simulink model "gtcs_math_v2"  (R2022b)
settings: Solver=VariableStepAuto  StartTime=0.0  StopTime=10  RelTol=1e-3
undefined symbols (not defined in the file or in its folder): B_load, B_motor, B_reducer, GearRatio, J_load, J_motor, J_reducer, ke, kt, L_motor, R_motor
libraries: slpidlib x1, simulink x1
settings Model: DataDictionary=gtcs_math_v1.sldd  Creator=yusuf.ogut  LastModifiedBy=Yusuf
settings ModelReferenceCC: EnableRefExpFcnMdlSchedulingChecks=on

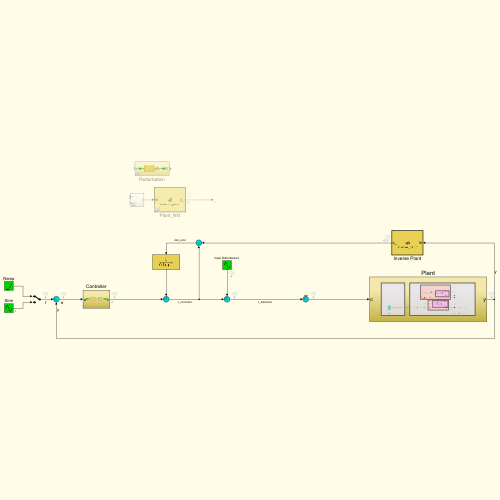
[thumbnail: Simulink's stored preview of the top-level diagram]
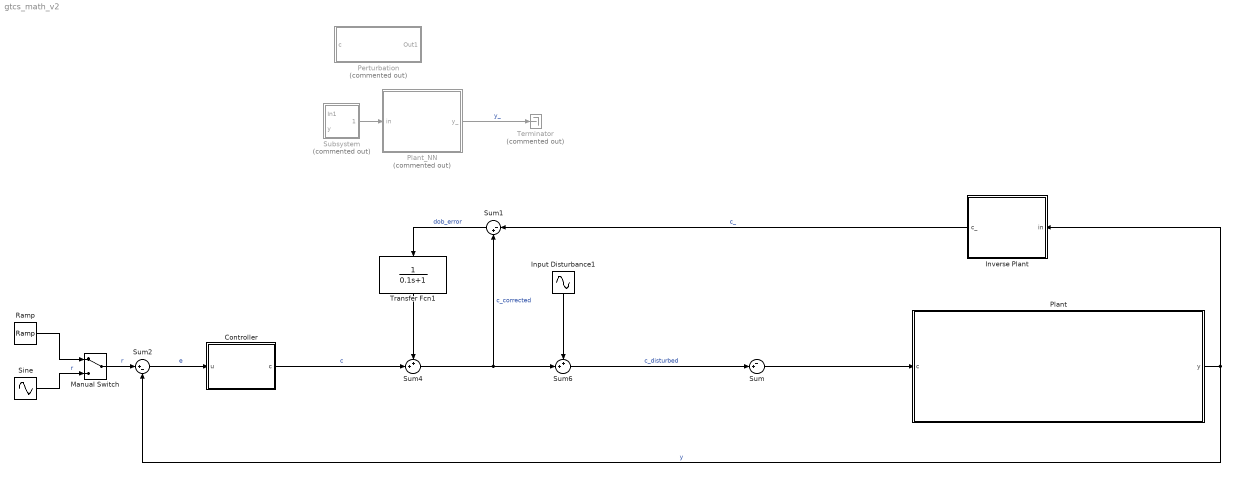
== system gtcs_math_v2 ==
  Controller : Subsystem
  Input Disturbance1 : Sin  SampleTime=0
  Inverse Plant : MATLAB Function  TreatAsAtomicUnit=on
  Manual Switch : ManualSwitch
  Perturbation : Subsystem  Commented=on
  Plant : Subsystem
  Plant_NN : MATLAB Function  Commented=on  TreatAsAtomicUnit=on
  Ramp : simulink/Sources/Ramp  slope=30  start=0  InitialOutput=0
  Sine : Sin  Amplitude=400  SampleTime=0
  Subsystem : Subsystem  Commented=on
  Sum : Sum  Inputs=-+|
  Sum1 : Sum  Inputs=|-+
  Sum2 : Sum  Inputs=|+-
  Sum4 : Sum  Inputs=++|
  Sum6 : Sum  Inputs=++|
  Terminator : Terminator  Commented=on
  Transfer Fcn1 : TransferFcn  Denominator=[0.1 1]
  wires:
  Plant/1(y) -> Inverse Plant/1(in), Sum2/2  "y"
  Sum2/1 -> Controller/1(u)  "e"
  Plant_NN/1(y_) -> Terminator/1  "y_"
  Sum/1 -> Plant/1(c)
  Sum6/1 -> Sum/2  "c_disturbed"
  Sine/1 -> Manual Switch/2  "r"
  Ramp/1 -> Manual Switch/1
  Manual Switch/1 -> Sum2/1  "r"
  Subsystem/1(Out1) -> Plant_NN/1(in)
  Controller/1(c) -> Sum4/2  "c"
  Sum4/1 -> Sum6/2, Sum1/2  "c_corrected"
  Input Disturbance1/1 -> Sum6/1
  Inverse Plant/1(c_) -> Sum1/1  "c_"
  Sum1/1 -> Transfer Fcn1/1  "dob_error"
  Transfer Fcn1/1 -> Sum4/1

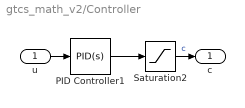
== system gtcs_math_v2/Controller ==
  u : Inport
  PID Controller1 : slpidlib/PID Controller  Controller=PID  Form=Parallel  TimeDomain=Continuous-time  UseExternalTs=off  SampleTime=-1  IntegratorMethod=Forward Euler  FilterMethod=Forward Euler  ControllerParametersSource=internal  P=1  I=0.12  UseKiTs=off  D=0  N=100  UseFilter=on  TunerSelectOption=Transfer Function Based (PID Tuner App)  InitialConditionSource=internal  InitialConditionForIntegrator=0  InitialConditionForFilter=0  DifferentiatorICPrevScaledInput=0  ExternalReset=none  TrackingMode=off  Kt=1  LimitOutput=off  SatLimitsSource=internal  UpperSaturationLimit=inf  LowerSaturationLimit=-inf  LinearizeAsGain=on  AntiWindupMode=none  Kb=1  LimitIntegrator=off  UpperIntegratorSaturationLimit=inf  LowerIntegratorSaturationLimit=-inf  POutMin=[]  POutMax=[]  IOutMin=[]  IOutMax=[]  DOutMin=[]  DOutMax=[]  NOutMin=[]  NOutMax=[]  SumOutMin=[]  SumOutMax=[]  SaturationOutMin=[]  SaturationOutMax=[]  PParamMin=[]  PParamMax=[]  IParamMin=[]  IParamMax=[]  DParamMin=[]  DParamMax=[]  NParamMin=[]  NParamMax=[]  KbParamMin=[]  KbParamMax=[]  KtParamMin=[]  KtParamMax=[]  KbOutMin=[]  KbOutMax=[]  KtOutMin=[]  KtOutMax=[]  IntegratorOutMin=[]  IntegratorOutMax=[]  FilterOutMin=[]  FilterOutMax=[]  SumI1OutMin=[]  SumI1OutMax=[]  SumI2OutMin=[]  SumI2OutMax=[]  SumI3OutMin=[]  SumI3OutMax=[]  SumI4OutMin=[]  SumI4OutMax=[]  SumDOutMin=[]  SumDOutMax=[]  DifferentiatorOutMin=[]  DifferentiatorOutMax=[]  FilterDiffOutCoefMin=[]  FilterDiffOutCoefMax=[]  ReciprocalOutMin=[]  ReciprocalOutMax=[]  SumDenOutMin=[]  SumDenOutMax=[]  SumNumOutMin=[]  SumNumOutMax=[]  DivideOutMin=[]  DivideOutMax=[]  UdiffTsProdOutMin=[]  UdiffTsProdOutMax=[]  NTsProdOutMin=[]  NTsProdOutMax=[]  UintegralTsProdOutMin=[]  UintegralTsProdOutMax=[]  UngainTsProdOutMin=[]  UngainTsProdOutMax=[]  ClampingZeroOutDataTypeStr=Inherit: Inherit via back propagation  ClampingZeroOutMin=[]  ClampingZeroOutMax=[]  FilterDenConstantOutDataTypeStr=Inherit: Inherit via back propagation  FilterDenConstantOutMin=[]  FilterDenConstantOutMax=[]  PCopyOutDataTypeStr=Inherit: Inherit via back propagation  PCopyOutMin=[]  PCopyOutMax=[]  NCopyOutDataTypeStr=Inherit: Inherit via back propagation  NCopyOutMin=[]  NCopyOutMax=[]  IntegratorContinuousStateAttributes=''  IntegratorStateMustResolveToSignalObject=off  IntegratorRTWStateStorageClass=Auto  FilterContinuousStateAttributes=''  FilterStateMustResolveToSignalObject=off  FilterRTWStateStorageClass=Auto  ParallelPVariant=InternalParameters  IdealPVariant=Disabled  IVariant=InternalParameters  DVariant=InternalParameters  IntegratorVariant=Continuous  SatVariant=Disabled  AWVariant=Passthrough  PCopyVariant=Disabled  TRVariant=Disabled  FdbkBlocksVariant=Forward  IdealPFdbkVariant=Disabled  SatFdbkVariant=Disabled  DerivativeFilterVariant=ContFilter  NVariant=InternalParameters  NCopyVariant=Disabled  FilterICVariant=InternalICsFilter  IntegratorICVariant=InternalICs  ExternalResetVariant=Disabled  TRSumVariant=Passthrough  SumFdbkVariant=Disabled  SumVariant=Sum_PID  TsampFilterVariant=InternalTs  TsampNgainVariant=Passthrough  TsampIntegralVariant=Passthrough  ExternalSaturationOutDataTypeStr=Inherit: Same as second input
  Saturation2 : Saturate  UpperLimit=28  LowerLimit=-28
  c : Outport
  wires:
  Saturation2/1 -> c/1  "c"
  PID Controller1/1 -> Saturation2/1
  u/1 -> PID Controller1/1

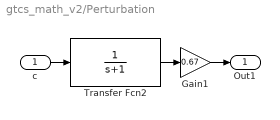
== system gtcs_math_v2/Perturbation ==
  c : Inport
  Gain1 : Gain  Gain=0.67
  Transfer Fcn2 : TransferFcn  Denominator=[1 1]
  Out1 : Outport
  wires:
  Gain1/1 -> Out1/1
  c/1 -> Transfer Fcn2/1
  Transfer Fcn2/1 -> Gain1/1

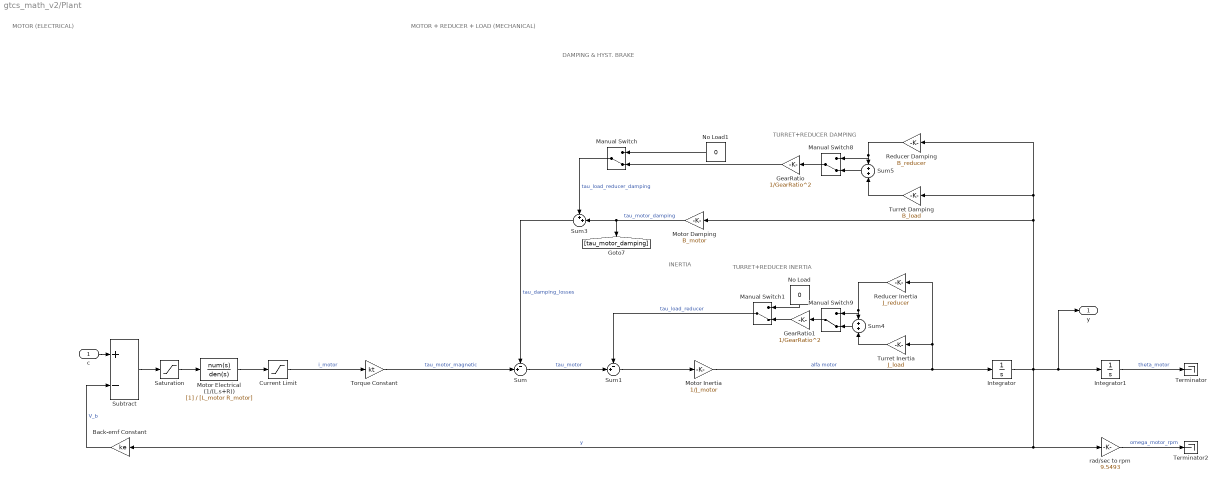
== system gtcs_math_v2/Plant ==
  note: TURRET+REDUCER INERTIA
  note: TURRET+REDUCER DAMPING
  note: DAMPING & HYST. BRAKE
  note: INERTIA
  note: MOTOR (ELECTRICAL)
  note: MOTOR + REDUCER + LOAD (MECHANICAL)
  c : Inport
  Back-emf Constant : Gain  Gain=ke
  Current Limit : Saturate  UpperLimit=80  LowerLimit=-80
  GearRatio : Gain  Gain=1/GearRatio^2
  GearRatio1 : Gain  Gain=1/GearRatio^2
  Integrator : Integrator
  Integrator1 : Integrator
  Manual Switch{,1,8..9} (4 alike) : ManualSwitch  CurrentSetting=0
  Motor Damping : Gain  Gain=B_motor
  Motor Electrical (1/(L.s+R)) : TransferFcn  Denominator=[L_motor R_motor]
  Motor Inertia : Gain  Gain=1/J_motor
  No Load : Constant  Value=0
  No Load1 : Constant  Value=0
  Reducer Damping : Gain  Gain=B_reducer
  Reducer Inertia : Gain  Gain=J_reducer
  Saturation : Saturate  UpperLimit=28  LowerLimit=-28
  Subtract : Sum  Inputs=+-
  Sum : Sum  Inputs=-+|
  Sum1 : Sum  Inputs=-+|
  Sum3 : Sum  Inputs=++|
  Sum4 : Sum
  Sum5 : Sum
  Terminator : Terminator
  Terminator2 : Terminator
  Torque Constant : Gain  Gain=kt
  Turret Damping : Gain  Gain=B_load
  Turret Inertia : Gain  Gain=J_load
  rad/sec to rpm : Gain  Gain=9.5493
  y : Outport
  wires:
  No Load/1 -> Manual Switch1/1
  Turret Damping/1 -> Sum5/2
  Reducer Inertia/1 -> Manual Switch9/1, Sum4/1
  GearRatio1/1 -> Manual Switch1/2
  Torque Constant/1 -> Sum/2  "tau_motor_magnetic"
  Manual Switch/1 -> Sum3/1  "tau_load_reducer_damping"
  Integrator/1 -> y/1, Integrator1/1, rad/sec to rpm/1, Back-emf Constant/1, Turret Damping/1, Reducer Damping/1, Motor Damping/1  "y"
  Current Limit/1 -> Torque Constant/1  "i_motor"
  No Load1/1 -> Manual Switch/1
  Manual Switch9/1 -> GearRatio1/1
  Sum3/1 -> Sum/1  "tau_damping_losses"
  Motor Inertia/1 -> Integrator/1, Turret Inertia/1, Reducer Inertia/1  "alfa motor"
  Sum4/1 -> Manual Switch9/2
  Sum1/1 -> Motor Inertia/1
  Manual Switch1/1 -> Sum1/1  "tau_load_reducer"
  GearRatio/1 -> Manual Switch/2
  Integrator1/1 -> Terminator/1  "theta_motor"
  Turret Inertia/1 -> Sum4/2
  Manual Switch8/1 -> GearRatio/1
  Reducer Damping/1 -> Manual Switch8/1, Sum5/1
  Sum/1 -> Sum1/2  "tau_motor"
  Motor Damping/1 -> [tau_motor_damping], Sum3/2  "tau_motor_damping"
  Sum5/1 -> Manual Switch8/2
  Saturation/1 -> Motor Electrical (1/(L.s+R))/1
  Back-emf Constant/1 -> Subtract/2  "V_b"
  c/1 -> Subtract/1
  rad/sec to rpm/1 -> Terminator2/1  "omega_motor_rpm"
  Motor Electrical (1/(L.s+R))/1 -> Current Limit/1
  Subtract/1 -> Saturation/1

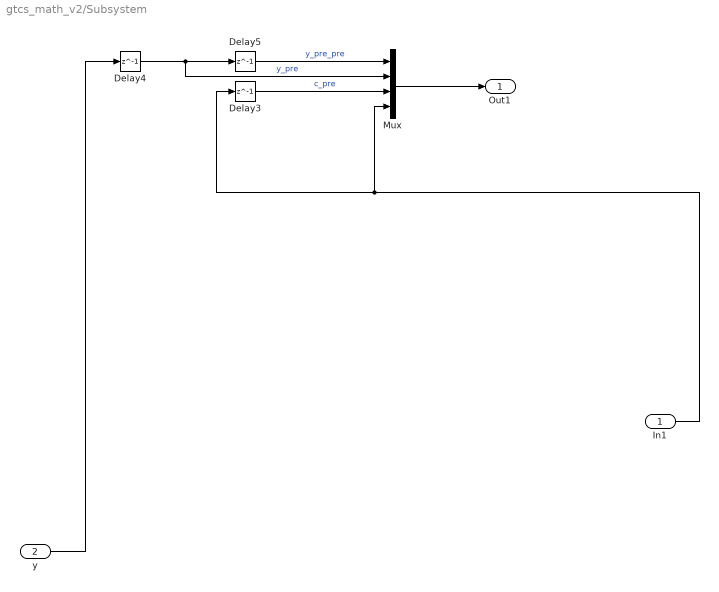
== system gtcs_math_v2/Subsystem ==
  In1 : Inport
  y : Inport  Port=2
  Delay3 : Delay  DelayLength=1  SampleTime=0.01
  Delay4 : Delay  DelayLength=1  SampleTime=0.01
  Delay5 : Delay  DelayLength=1  SampleTime=0.01
  Mux : Mux
  Out1 : Outport
  wires:
  In1/1 -> Mux/4, Delay3/1
  Delay4/1 -> Delay5/1, Mux/2  "y_pre"
  Delay3/1 -> Mux/3  "c_pre"
  Mux/1 -> Out1/1
  Delay5/1 -> Mux/1  "y_pre_pre"
  y/1 -> Delay4/1

== matlab function gtcs_math_v2/Inverse Plant ==
  data: in input; c_ output
function c_ = inverse_plant(in)
    y_ =  0.0534; r_ = 16.0258;
    c__ = 1.2811; r__ = 384.4721;
    input_training = (in - c__)/r__;
    Phi = [ -0.7229   -0.1132         0         0
            -0.7229   -0.1132         0         0
            -0.7229   -0.1132         0         0
            -0.4882   -0.4882   -0.4882   -0.1223];
    BIAS = -.1;
    % FORWARD PASS:
    NUM_INP = 1; NUM_HID = 3;
    input_vector = [input_training;BIAS];
    S1 = Phi(1:NUM_HID,1:NUM_INP+1)*input_vector;
    O1 = tanh(S1);
    S2 = Phi(NUM_HID+1:end,1:NUM_HID+1)*[O1;BIAS];
    c_ = S2*r_+y_;
end

== matlab function gtcs_math_v2/Plant_NN ==
  data: in input; y_ output
function y_ = forward_pass(in)
    c_sf_i_4 = 24.3519;     r_sf_i_4 = 3.6481;
    c_sf_i_3 = 14;          r_sf_i_3 = 14;
    c_sf_i_2 = 249.4384;    r_sf_i_2 = 249.4384;
    c_sf_i_1 = 249.4394;    r_sf_i_1 = 249.4394;
    c_sf_o_1 = 249.3494;    r_sf_o_1 = 249.4394;
    input_training = (([in(4) in(3) in(2) in(1)] - [c_sf_i_4 c_sf_i_3 c_sf_i_2 c_sf_i_1]) ./ [r_sf_i_4 r_sf_i_3 r_sf_i_2 r_sf_i_1])';

    Phi = [     0.0386   -0.0713   -0.3476   -0.3525    0.0122         0         0         0         0         0         0
                0.0386   -0.0713   -0.3476   -0.3525    0.0122         0         0         0         0         0         0
                0.0386   -0.0713   -0.3476   -0.3525    0.0122         0         0         0         0         0         0
                0.0386   -0.0713   -0.3476   -0.3525    0.0122         0         0         0         0         0         0
                0.0386   -0.0713   -0.3476   -0.3525    0.0122         0         0         0         0         0         0
                0.0386   -0.0713   -0.3476   -0.3525    0.0122         0         0         0         0         0         0
                0.0386   -0.0713   -0.3476   -0.3525    0.0122         0         0         0         0         0         0
                0.0386   -0.0713   -0.3476   -0.3525    0.0122         0         0         0         0         0         0
                0.0386   -0.0713   -0.3476   -0.3525    0.0122         0         0         0         0         0         0
                0.0386   -0.0713   -0.3476   -0.3525    0.0122         0         0         0         0         0         0
               -0.1525   -0.1525   -0.1525   -0.1525   -0.1525   -0.1525   -0.1525   -0.1525   -0.1525   -0.1525   -0.1037];
    BIAS = -.1;
    % FORWARD PASS:
    NUM_INP = 4; NUM_HID = 10;
    input_vector = [input_training;BIAS];
    S1 = Phi(1:NUM_HID,1:NUM_INP+1)*input_vector;
    O1 = tanh(S1);
    S2 = Phi(NUM_HID+1:end,1:NUM_HID+1)*[O1;BIAS];
    y_ = S2 * r_sf_o_1 + c_sf_o_1;
end
